simulink model "q1_3"  (Simulink 7.8)
settings: Solver=ode45  StartTime=0.0  StopTime=10.0  RelTol=1e-3
settings Model: Creator=narmada_hm  LastModifiedBy=Dan
settings DebuggingCC: InitInArrayFormatMsg=none
settings GRTTargetCC: CombineOutputUpdateFcns=on

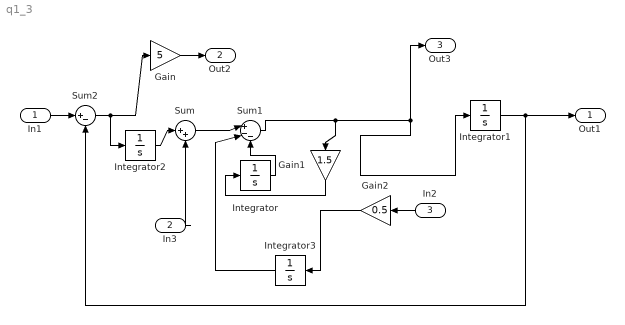
== system q1_3 ==
  In1 : Inport
  In3 : Inport  Port=2
  In2 : Inport  Port=3
  Gain : Gain  Gain=5
  Gain1 : Gain  Gain=1.5
  Gain2 : Gain  Gain=0.5
  Integrator{,1..3} (4 alike) : Integrator
  Sum : Sum  Inputs=|++
  Sum1 : Sum  Inputs=|+--
  Sum2 : Sum  Inputs=|+-
  Out1 : Outport
  Out2 : Outport  Port=2
  Out3 : Outport  Port=3
  wires:
  Sum1/1 -> Out3/1, Integrator1/1, Gain1/1
  In3/1 -> Sum/2
  Gain/1 -> Out2/1
  In1/1 -> Sum2/1
  Sum2/1 -> Gain/1, Integrator2/1
  Integrator2/1 -> Sum/1
  Sum/1 -> Sum1/1
  Integrator1/1 -> Sum2/2, Out1/1
  Gain1/1 -> Integrator/1
  In2/1 -> Gain2/1
  Gain2/1 -> Integrator3/1
  Integrator/1 -> Sum1/3
  Integrator3/1 -> Sum1/2
